simulink model "DCmotor"  (Simulink 8.5)
settings: Solver=ode45  StartTime=0.0  StopTime=10.0  RelTol=1e-3
values from neighbouring files (symbols this model uses):
  c = 8    [Ninad_deshpande_DCmotordata.m]
  I = 2    [Ninad_deshpande_DCmotordata.m]
  KT = 0.12    [Ninad_deshpande_DCmotordata.m]
  KV = 0.127    [Ninad_deshpande_DCmotordata.m]
  L = 0.01    [Ninad_deshpande_DCmotordata.m]
  R = 0.053    [Ninad_deshpande_DCmotordata.m]
  v = 48    [Ninad_deshpande_DCmotordata.m]
settings Model: Creator=lenovo  LastModifiedBy=lenovo
settings DataIOCC: SignalLoggingSaveFormat=Dataset
settings OptimizationCC: ExpressionDepthLimit=128
settings DebuggingCC: UnderspecifiedInitializationDetection=Simplified  MergeDetectMultiDrivingBlocksExec=error  FcnCallInpInsideContextMsg=EnableAllAsError  StateNameClashWarn=none
settings GRTTargetCC: CombineOutputUpdateFcns=on  GRTInterface=off

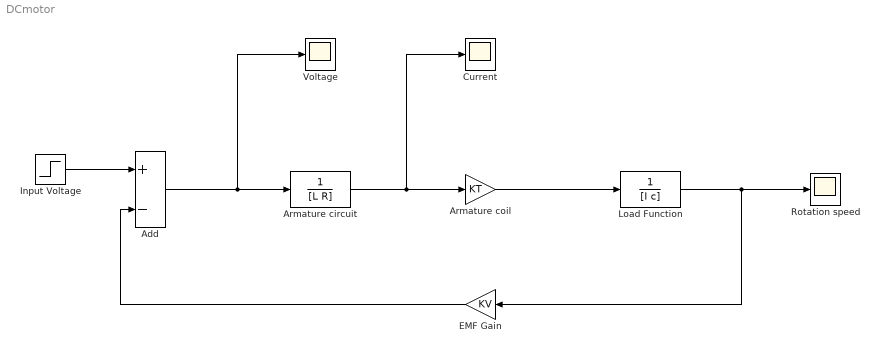
== system DCmotor ==
  Add : Sum  Inputs=+-
  Armature circuit : TransferFcn  Denominator=[L R]
  Armature coil : Gain  Gain=KT
  Current : Scope
  EMF Gain : Gain  Gain=KV
  Input Voltage : Step  After=v  SampleTime=0
  Load Function : TransferFcn  Denominator=[I c]
  Rotation speed : Scope
      settings: SaveName=ScopeData2
  Voltage : Scope
  wires:
  Input Voltage/1 -> Add/1
  Armature coil/1 -> Load Function/1
  Armature circuit/1 -> Current/1, Armature coil/1
  Add/1 -> Voltage/1, Armature circuit/1
  Load Function/1 -> EMF Gain/1, Rotation speed/1
  EMF Gain/1 -> Add/2
